simulink model "DrivetrainEv_3motor_VDBS"  (R2020a)
settings: configuration reference "Reference" (kept outside this file)
undefined symbols (not defined in the file): b, F0z, h, k, Ndiff_rear, VEH
libraries: vehdynlibsuspension x9, vehdynlibtire x8, autolibsharedcoupling x4, autolibcoupling x2, autolibutils x2, sharedtransform x2, autolibshareddiff x1, autolibshared x1, vehdynlibeom x1, vehdynlibtirecommon x1, vehdynlibsteering x1
(part 1 of 5)
settings Model: DataDictionary=System_Data_Dictionary.sldd  ModifiedByFormat=The MathWorks, Inc.  PauseTimes=10  OrderedModelArguments=off  Creator=The MathWorks, Inc.  LastModifiedBy=The MathWorks, Inc.
settings ConfigSetRef: SourceName=Reference

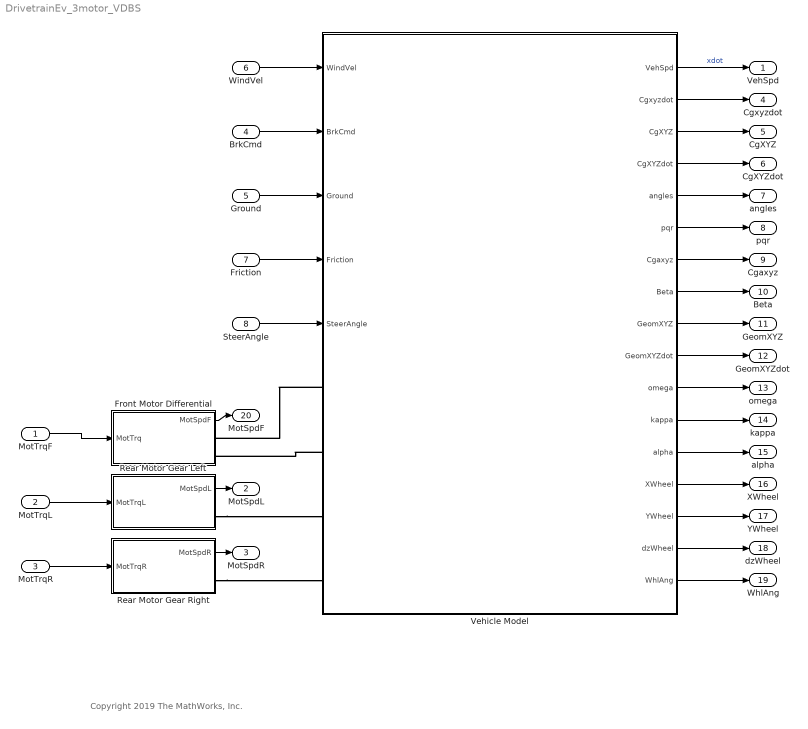
== system DrivetrainEv_3motor_VDBS ==
  note: Copyright 2019 The MathWorks, Inc.
  MotTrqF : Inport
  MotTrqL : Inport  Port=2
  MotTrqR : Inport  Port=3
  BrkCmd : Inport  Port=4
  Ground : Inport  Port=5
  WindVel : Inport  Port=6
  Friction : Inport  Port=7
  SteerAngle : Inport  Port=8
  Front Motor Differential : Subsystem  VariantControl=0
  Rear Motor Gear Left : Subsystem  VariantControl=0
  Rear Motor Gear Right : Subsystem  VariantControl=0
  Vehicle Model : Subsystem
  VehSpd : Outport  VectorParamsAs1DForOutWhenUnconnected=off
  MotSpdL : Outport  Port=2  VectorParamsAs1DForOutWhenUnconnected=off  BusOutputAsStruct=on
  MotSpdR : Outport  Port=3  VectorParamsAs1DForOutWhenUnconnected=off  BusOutputAsStruct=on
  Cgxyzdot : Outport  Port=4  VectorParamsAs1DForOutWhenUnconnected=off
  CgXYZ : Outport  Port=5  VectorParamsAs1DForOutWhenUnconnected=off
  CgXYZdot : Outport  Port=6  VectorParamsAs1DForOutWhenUnconnected=off
  angles : Outport  Port=7  VectorParamsAs1DForOutWhenUnconnected=off
  pqr : Outport  Port=8  VectorParamsAs1DForOutWhenUnconnected=off
  Cgaxyz : Outport  Port=9  VectorParamsAs1DForOutWhenUnconnected=off
  Beta : Outport  Port=10  VectorParamsAs1DForOutWhenUnconnected=off
  GeomXYZ : Outport  Port=11  VectorParamsAs1DForOutWhenUnconnected=off
  GeomXYZdot : Outport  Port=12  VectorParamsAs1DForOutWhenUnconnected=off
  omega : Outport  Port=13  PortDimensions=4  VectorParamsAs1DForOutWhenUnconnected=off
  kappa : Outport  Port=14  PortDimensions=4  VectorParamsAs1DForOutWhenUnconnected=off
  alpha : Outport  Port=15  PortDimensions=4  VectorParamsAs1DForOutWhenUnconnected=off
  XWheel : Outport  Port=16  VectorParamsAs1DForOutWhenUnconnected=off
  YWheel : Outport  Port=17  VectorParamsAs1DForOutWhenUnconnected=off
  dzWheel : Outport  Port=18  VectorParamsAs1DForOutWhenUnconnected=off
  WhlAng : Outport  Port=19  VectorParamsAs1DForOutWhenUnconnected=off
  MotSpdF : Outport  Port=20  VectorParamsAs1DForOutWhenUnconnected=off  BusOutputAsStruct=on
  wires:
  Rear Motor Gear Left/1(MotSpdL) -> MotSpdL/1
  Vehicle Model/12(kappa) -> kappa/1
  Vehicle Model/13(alpha) -> alpha/1
  Ground/1 -> Vehicle Model/3(Ground)
  Vehicle Model/14(XWheel) -> XWheel/1
  WindVel/1 -> Vehicle Model/1(WindVel)
  Vehicle Model/5(angles) -> angles/1
  Friction/1 -> Vehicle Model/4(Friction)
  SteerAngle/1 -> Vehicle Model/5(SteerAngle)
  Vehicle Model/8(Beta) -> Beta/1
  Vehicle Model/15(YWheel) -> YWheel/1
  Vehicle Model/17(WhlAng) -> WhlAng/1
  Vehicle Model/1(VehSpd) -> VehSpd/1  "xdot"
  Vehicle Model/10(GeomXYZdot) -> GeomXYZdot/1
  Vehicle Model/2(Cgxyzdot) -> Cgxyzdot/1
  Vehicle Model/4(CgXYZdot) -> CgXYZdot/1
  Vehicle Model/3(CgXYZ) -> CgXYZ/1
  Vehicle Model/7(Cgaxyz) -> Cgaxyz/1
  Vehicle Model/11(omega) -> omega/1
  Vehicle Model/9(GeomXYZ) -> GeomXYZ/1
  BrkCmd/1 -> Vehicle Model/2(BrkCmd)
  Vehicle Model/16(dzWheel) -> dzWheel/1
  Vehicle Model/6(pqr) -> pqr/1
  MotTrqL/1 -> Rear Motor Gear Left/1(MotTrqL)
  Rear Motor Gear Right/1(MotSpdR) -> MotSpdR/1
  MotTrqR/1 -> Rear Motor Gear Right/1(MotTrqR)
  Front Motor Differential/1(MotSpdF) -> MotSpdF/1
  MotTrqF/1 -> Front Motor Differential/1(MotTrq)
  connections:
  Vehicle Model/LConn1 -- Front Motor Differential/RConn1
  Vehicle Model/LConn2 -- Front Motor Differential/RConn2
  Rear Motor Gear Left/RConn1 -- Vehicle Model/LConn3
  Rear Motor Gear Right/RConn1 -- Vehicle Model/LConn4

== system DrivetrainEv_3motor_VDBS/Front Motor Differential ==
  MotTrq : Inport
  Axle Compliance : autolibsharedcoupling/Torsional Compliance  port_config=Two-way connection  extInfo=off  k=k  b=b  theta_o=theta_o  domega_o=domega_o  omega_c=omega_c  blkID=0  aMode=1
      settings: SourceProductName=Powertrain Blockset
  Axle Compliance1 : autolibsharedcoupling/Torsional Compliance  port_config=Two-way connection  extInfo=off  k=k  b=b  theta_o=theta_o  domega_o=domega_o  omega_c=omega_c  blkID=0  aMode=1
      settings: SourceProductName=Powertrain Blockset
  Open Differential : autolibshareddiff/Open Differential  DiffEffModelPopup=Constant  InterpMethod=Linear point-slope  extTamb=off  shaftSwitchMask=To the left of center-line  Ndiff=Ndiff_front  Jd=Jd  bd=bd  Jw1=Jw1  bw1=bw1  Jw2=Jw2  bw2=bw2  omegaw1o=omegaw1o  omegaw2o=omegaw2o  eta=1  eta_tbl=reshape([0.64 0.76 0.8 0.81 0.83 0.84 0.84 0.56 0.73 0.78 0.8 0.83 0.84 0.84 0.54 0.71 0.77 0.8 0.82 0.84 0.84 0.53 0.71 0.77 0.8 0.83 0.84 0.84 0.51 0.71 0.77 0.8 0.83 0.84 0.85 0.52 0.7 0.77 0.8 0.83 0.84 0.85 0.51 0.71 0.76 0.79 0.83 0.84 0.85 0.5 0.69 0.76 0.79 0.82 0.84 0.85 0.45 0.68 0.75 0.78 0.82 0.84 0.85 0.43 0.67 0.74 0.78 0.81 0.83 0.84 0.38 0.63 0.71 0.75 0.8 0.82 0.83 0.81 0.86 0.88 0.89 0.89 0.89 0.9 0.77 0.85 0.87 0.88 0.89 0.9 0.9 0.72 0.82 0.86 0.87 0.88 0.89 0.9 0.68 0.8 0.84 0.86 0.88 0.89 0.89 0.67 0.8 0.84 0.86 0.88 0.89 0.9 0.67 0.8 0.84 0.86 0.88 0.89 0.9 0.65 0.8 0.84 0.86 0.88 0.89 0.9 0.64 0.79 0.83 0.86 0.88 0.89 0.9 0.63 0.78 0.83 0.86 0.88 0.89 0.9 0.59 0.76 0.82 0.85 0.87 0.89 0.9 0.53 0.73 0.8 0.83 0.86 0.88 0.89], 7, 11, 2)  Trq_bpts=[25, 50, 75, 100, 150, 200, 250]  omega_bpts=[52.4 78.5 105 131 157 183 209 262 314 419 524]  Temp_bpts=[290 358]  Tamb=297.15  maxAbsSpd=5e3  aMode=1
      settings: SourceProductName=Powertrain Blockset
  Terminator6 : Terminator
  Two-Way Connection1 : TwoWayConnection
  Two-Way Connection3 : TwoWayConnection
  A1 : PMIOPort  Side=Right
  A2 : PMIOPort  Port=2  Side=Right
  MotSpdF : Outport  VectorParamsAs1DForOutWhenUnconnected=off
  wires:
  Open Differential/2 -> MotSpdF/1  "MotSpdF"
  Open Differential/4 -> Two-Way Connection3/1
  Open Differential/3 -> Two-Way Connection1/1
  Two-Way Connection1/1 -> Open Differential/2
  Open Differential/1 -> Terminator6/1  "Diff"
  Two-Way Connection3/1 -> Open Differential/3
  MotTrq/1 -> Open Differential/1
  connections:
  Axle Compliance/LConn1 -- Two-Way Connection1/RConn1
  Axle Compliance/RConn1 -- A1/RConn1
  Axle Compliance1/LConn1 -- Two-Way Connection3/RConn1
  A2/RConn1 -- Axle Compliance1/RConn1

== system DrivetrainEv_3motor_VDBS/Rear Motor Gear Left ==
  MotTrqL : Inport
  Axle Compliance : autolibsharedcoupling/Torsional Compliance  port_config=Two-way connection  extInfo=off  k=k  b=b  theta_o=theta_o  domega_o=domega_o  omega_c=omega_c  blkID=0  aMode=1
      settings: SourceProductName=Powertrain Blockset
  Gearbox : autolibcoupling/Gearbox  port_config=Simulink  input_config=Torque input - velocity output  DiffEffModelPopup=Constant  InterpMethod=Flat  dirSwitch=on  extTamb=off  N=Ndiff_rear  J1=J1  J2=J2  b1=b1_g  b2=b2_g  theta1_o=0  w1_o=w1_o  eta=1  eta_tbl=reshape([0.64 0.76 0.8 0.81 0.83 0.84 0.84 0.56 0.73 0.78 0.8 0.83 0.84 0.84 0.54 0.71 0.77 0.8 0.82 0.84 0.84 0.53 0.71 0.77 0.8 0.83 0.84 0.84 0.51 0.71 0.77 0.8 0.83 0.84 0.85 0.52 0.7 0.77 0.8 0.83 0.84 0.85 0.51 0.71 0.76 0.79 0.83 0.84 0.85 0.5 0.69 0.76 0.79 0.82 0.84 0.85 0.45 0.68 0.75 0.78 0.82 0.84 0.85 0.43 0.67 0.74 0.78 0.81 0.83 0.84 0.38 0.63 0.71 0.75 0.8 0.82 0.83 0.81 0.86 0.88 0.89 0.89 0.89 0.9 0.77 0.85 0.87 0.88 0.89 0.9 0.9 0.72 0.82 0.86 0.87 0.88 0.89 0.9 0.68 0.8 0.84 0.86 0.88 0.89 0.89 0.67 0.8 0.84 0.86 0.88 0.89 0.9 0.67 0.8 0.84 0.86 0.88 0.89 0.9 0.65 0.8 0.84 0.86 0.88 0.89 0.9 0.64 0.79 0.83 0.86 0.88 0.89 0.9 0.63 0.78 0.83 0.86 0.88 0.89 0.9 0.59 0.76 0.82 0.85 0.87 0.89 0.9 0.53 0.73 0.8 0.83 0.86 0.88 0.89], 7, 11, 2)  Trq_bpts=[25, 50, 75, 100, 150, 200, 250]  omega_bpts=[52.4 78.5 105 131 157 183 209 262 314 419 524]  Temp_bpts=[290 358]  Tamb=297.15  blkID=0
      settings: SourceProductBaseCode=PW
  Terminator6 : Terminator
  Two-Way Connection1 : TwoWayConnection
  AL : PMIOPort  Side=Right
  MotSpdL : Outport  VectorParamsAs1DForOutWhenUnconnected=off
  wires:
  Gearbox/2 -> MotSpdL/1
  MotTrqL/1 -> Gearbox/1
  Gearbox/3 -> Two-Way Connection1/1
  Two-Way Connection1/1 -> Gearbox/2
  Gearbox/1 -> Terminator6/1
  connections:
  Axle Compliance/LConn1 -- Two-Way Connection1/RConn1
  AL/RConn1 -- Axle Compliance/RConn1

== system DrivetrainEv_3motor_VDBS/Rear Motor Gear Right ==
  MotTrqR : Inport
  Axle Compliance : autolibsharedcoupling/Torsional Compliance  port_config=Two-way connection  extInfo=off  k=k  b=b  theta_o=theta_o  domega_o=domega_o  omega_c=omega_c  blkID=0  aMode=1
      settings: SourceProductName=Powertrain Blockset
  Gearbox : autolibcoupling/Gearbox  port_config=Simulink  input_config=Torque input - velocity output  DiffEffModelPopup=Constant  InterpMethod=Flat  dirSwitch=on  extTamb=off  N=Ndiff_rear  J1=J1  J2=J2  b1=b1_g  b2=b2_g  theta1_o=0  w1_o=w1_o  eta=1  eta_tbl=reshape([0.64 0.76 0.8 0.81 0.83 0.84 0.84 0.56 0.73 0.78 0.8 0.83 0.84 0.84 0.54 0.71 0.77 0.8 0.82 0.84 0.84 0.53 0.71 0.77 0.8 0.83 0.84 0.84 0.51 0.71 0.77 0.8 0.83 0.84 0.85 0.52 0.7 0.77 0.8 0.83 0.84 0.85 0.51 0.71 0.76 0.79 0.83 0.84 0.85 0.5 0.69 0.76 0.79 0.82 0.84 0.85 0.45 0.68 0.75 0.78 0.82 0.84 0.85 0.43 0.67 0.74 0.78 0.81 0.83 0.84 0.38 0.63 0.71 0.75 0.8 0.82 0.83 0.81 0.86 0.88 0.89 0.89 0.89 0.9 0.77 0.85 0.87 0.88 0.89 0.9 0.9 0.72 0.82 0.86 0.87 0.88 0.89 0.9 0.68 0.8 0.84 0.86 0.88 0.89 0.89 0.67 0.8 0.84 0.86 0.88 0.89 0.9 0.67 0.8 0.84 0.86 0.88 0.89 0.9 0.65 0.8 0.84 0.86 0.88 0.89 0.9 0.64 0.79 0.83 0.86 0.88 0.89 0.9 0.63 0.78 0.83 0.86 0.88 0.89 0.9 0.59 0.76 0.82 0.85 0.87 0.89 0.9 0.53 0.73 0.8 0.83 0.86 0.88 0.89], 7, 11, 2)  Trq_bpts=[25, 50, 75, 100, 150, 200, 250]  omega_bpts=[52.4 78.5 105 131 157 183 209 262 314 419 524]  Temp_bpts=[290 358]  Tamb=297.15  blkID=0
      settings: SourceProductBaseCode=PW
  Terminator6 : Terminator
  Two-Way Connection1 : TwoWayConnection
  AR : PMIOPort  Side=Right
  MotSpdR : Outport  VectorParamsAs1DForOutWhenUnconnected=off
  wires:
  Gearbox/1 -> Terminator6/1
  Two-Way Connection1/1 -> Gearbox/2
  Gearbox/3 -> Two-Way Connection1/1
  MotTrqR/1 -> Gearbox/1
  Gearbox/2 -> MotSpdR/1
  connections:
  AR/RConn1 -- Axle Compliance/RConn1
  Axle Compliance/LConn1 -- Two-Way Connection1/RConn1

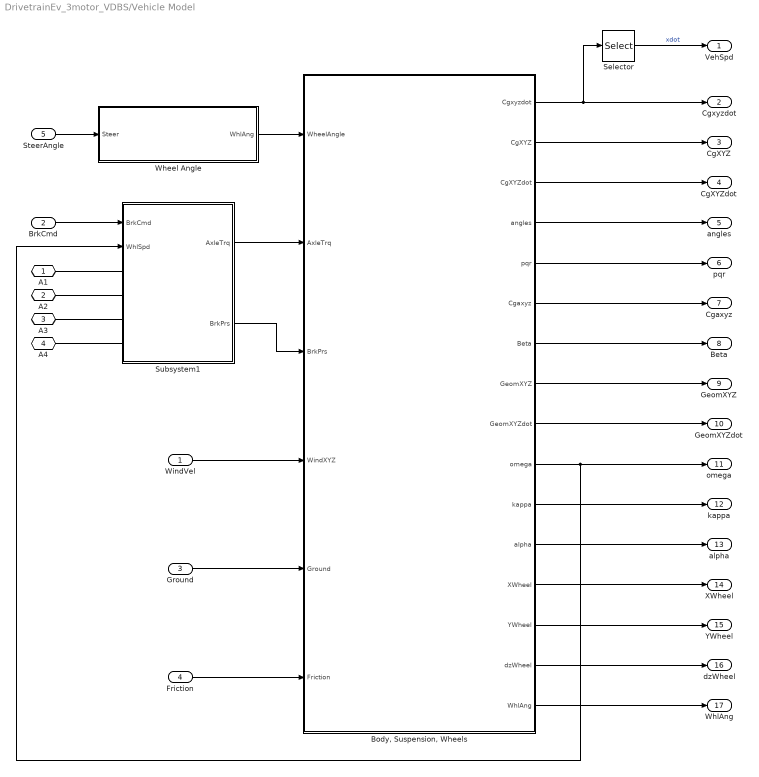
== system DrivetrainEv_3motor_VDBS/Vehicle Model ==
  WindVel : Inport
  BrkCmd : Inport  Port=2
  Ground : Inport  Port=3
  Friction : Inport  Port=4
  SteerAngle : Inport  Port=5
  "Body, Suspension, Wheels" : Subsystem  Variant=on  VariantControlMode=Label  LabelModeActiveChoice=1
  Selector : Selector  InputPortWidth=3  IndexOptions=Index vector (dialog)  Indices=1  OutputSizes=1
  Subsystem1 : Subsystem
  Wheel Angle : Subsystem
  A1 : PMIOPort  Side=Left
  A2 : PMIOPort  Port=2  Side=Left
  A3 : PMIOPort  Port=3  Side=Left
  A4 : PMIOPort  Port=4  Side=Left
  VehSpd : Outport  VectorParamsAs1DForOutWhenUnconnected=off
  Cgxyzdot : Outport  Port=2  VectorParamsAs1DForOutWhenUnconnected=off
  CgXYZ : Outport  Port=3  VectorParamsAs1DForOutWhenUnconnected=off
  CgXYZdot : Outport  Port=4  VectorParamsAs1DForOutWhenUnconnected=off
  angles : Outport  Port=5  VectorParamsAs1DForOutWhenUnconnected=off
  pqr : Outport  Port=6  VectorParamsAs1DForOutWhenUnconnected=off
  Cgaxyz : Outport  Port=7  VectorParamsAs1DForOutWhenUnconnected=off
  Beta : Outport  Port=8  VectorParamsAs1DForOutWhenUnconnected=off
  GeomXYZ : Outport  Port=9  VectorParamsAs1DForOutWhenUnconnected=off
  GeomXYZdot : Outport  Port=10  VectorParamsAs1DForOutWhenUnconnected=off
  omega : Outport  Port=11  PortDimensions=4  VectorParamsAs1DForOutWhenUnconnected=off
  kappa : Outport  Port=12  PortDimensions=4  VectorParamsAs1DForOutWhenUnconnected=off
  alpha : Outport  Port=13  PortDimensions=4  VectorParamsAs1DForOutWhenUnconnected=off
  XWheel : Outport  Port=14  VectorParamsAs1DForOutWhenUnconnected=off
  YWheel : Outport  Port=15  VectorParamsAs1DForOutWhenUnconnected=off
  dzWheel : Outport  Port=16  VectorParamsAs1DForOutWhenUnconnected=off
  WhlAng : Outport  Port=17  VectorParamsAs1DForOutWhenUnconnected=off
  wires:
  "Body, Suspension, Wheels"/10(omega) -> Subsystem1/2(WhlSpd), omega/1
  "Body, Suspension, Wheels"/8(GeomXYZ) -> GeomXYZ/1
  BrkCmd/1 -> Subsystem1/1(BrkCmd)
  "Body, Suspension, Wheels"/13(XWheel) -> XWheel/1
  "Body, Suspension, Wheels"/3(CgXYZdot) -> CgXYZdot/1
  "Body, Suspension, Wheels"/2(CgXYZ) -> CgXYZ/1
  "Body, Suspension, Wheels"/15(dzWheel) -> dzWheel/1
  "Body, Suspension, Wheels"/6(Cgaxyz) -> Cgaxyz/1
  "Body, Suspension, Wheels"/1(Cgxyzdot) -> Selector/1, Cgxyzdot/1
  "Body, Suspension, Wheels"/5(pqr) -> pqr/1
  "Body, Suspension, Wheels"/4(angles) -> angles/1
  "Body, Suspension, Wheels"/14(YWheel) -> YWheel/1
  "Body, Suspension, Wheels"/9(GeomXYZdot) -> GeomXYZdot/1
  "Body, Suspension, Wheels"/12(alpha) -> alpha/1
  "Body, Suspension, Wheels"/11(kappa) -> kappa/1
  "Body, Suspension, Wheels"/7(Beta) -> Beta/1
  "Body, Suspension, Wheels"/16(WhlAng) -> WhlAng/1
  Selector/1 -> VehSpd/1  "xdot"
  SteerAngle/1 -> Wheel Angle/1(Steer)
  WindVel/1 -> "Body, Suspension, Wheels"/4(WindXYZ)
  Wheel Angle/1(WhlAng) -> "Body, Suspension, Wheels"/1(WheelAngle)
  Ground/1 -> "Body, Suspension, Wheels"/5(Ground)
  Friction/1 -> "Body, Suspension, Wheels"/6(Friction)
  Subsystem1/2(BrkPrs) -> "Body, Suspension, Wheels"/3(BrkPrs)
  Subsystem1/1(AxleTrq) -> "Body, Suspension, Wheels"/2(AxleTrq)
  connections:
  Subsystem1/LConn1 -- A1/RConn1
  A2/RConn1 -- Subsystem1/LConn2
  A3/RConn1 -- Subsystem1/LConn3
  A4/RConn1 -- Subsystem1/LConn4

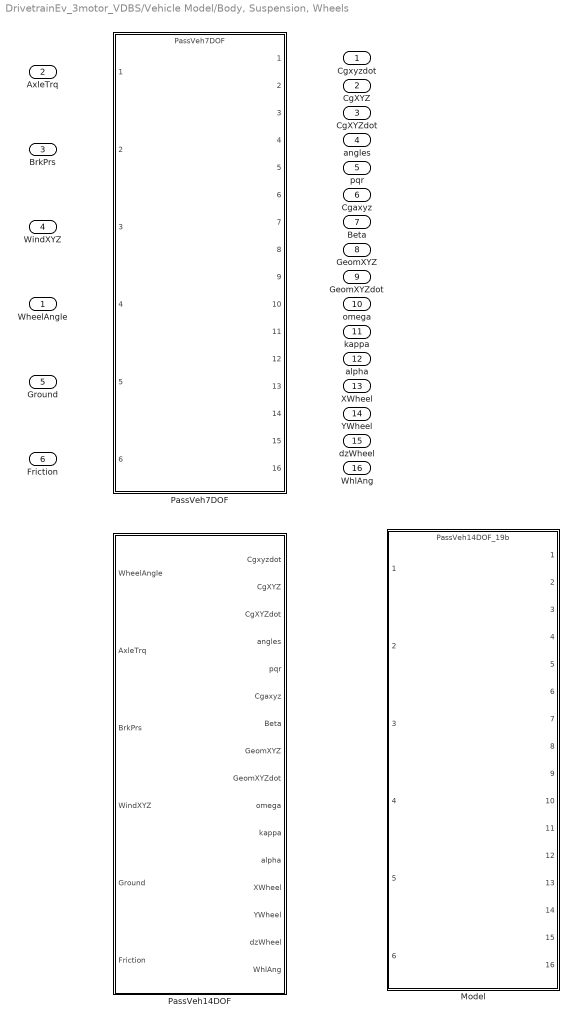
== system DrivetrainEv_3motor_VDBS/Vehicle Model/Body, Suspension, Wheels ==
  WheelAngle : Inport
  AxleTrq : Inport  Port=2
  BrkPrs : Inport  Port=3
  WindXYZ : Inport  Port=4
  Ground : Inport  Port=5
  Friction : Inport  Port=6
  Model : ModelReference  ModelNameDialog=PassVeh14DOF_19b.slx  SimulationMode=Normal  VariantControl=Choice  ModelReferenceVersion=1.318
  PassVeh14DOF : Subsystem  VariantControl=1
  PassVeh7DOF : ModelReference  DisableCoverage=on  ModelNameDialog=PassVeh7DOF  VariantControl=0  ModelReferenceVersion=1.140
  Cgxyzdot : Outport  VectorParamsAs1DForOutWhenUnconnected=off
  CgXYZ : Outport  Port=2  VectorParamsAs1DForOutWhenUnconnected=off
  CgXYZdot : Outport  Port=3  VectorParamsAs1DForOutWhenUnconnected=off
  angles : Outport  Port=4  VectorParamsAs1DForOutWhenUnconnected=off
  pqr : Outport  Port=5  VectorParamsAs1DForOutWhenUnconnected=off
  Cgaxyz : Outport  Port=6  VectorParamsAs1DForOutWhenUnconnected=off
  Beta : Outport  Port=7  VectorParamsAs1DForOutWhenUnconnected=off
  GeomXYZ : Outport  Port=8  VectorParamsAs1DForOutWhenUnconnected=off
  GeomXYZdot : Outport  Port=9  VectorParamsAs1DForOutWhenUnconnected=off
  omega : Outport  Port=10  PortDimensions=4  VectorParamsAs1DForOutWhenUnconnected=off
  kappa : Outport  Port=11  PortDimensions=4  VectorParamsAs1DForOutWhenUnconnected=off
  alpha : Outport  Port=12  PortDimensions=4  VectorParamsAs1DForOutWhenUnconnected=off
  XWheel : Outport  Port=13  VectorParamsAs1DForOutWhenUnconnected=off
  YWheel : Outport  Port=14  VectorParamsAs1DForOutWhenUnconnected=off
  dzWheel : Outport  Port=15  VectorParamsAs1DForOutWhenUnconnected=off
  WhlAng : Outport  Port=16  VectorParamsAs1DForOutWhenUnconnected=off

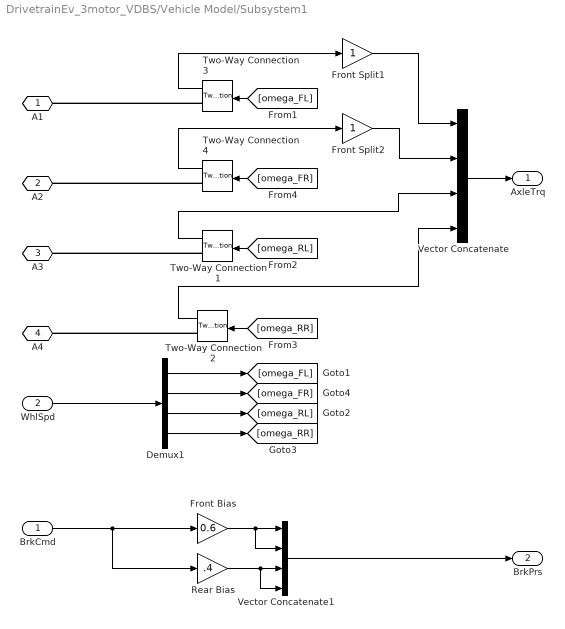
== system DrivetrainEv_3motor_VDBS/Vehicle Model/Subsystem1 ==
  BrkCmd : Inport
  WhlSpd : Inport  Port=2
  Demux1 : Demux
  Front Bias : Gain  Gain=0.6
  Front Split1 : Gain
  Front Split2 : Gain
  Rear Bias : Gain  Gain=.4
  Two-Way Connection{1..4} (4 alike) : TwoWayConnection
  Vector Concatenate : Concatenate  NumInputs=4
  Vector Concatenate1 : Concatenate  NumInputs=4
  A1 : PMIOPort  Side=Left
  A2 : PMIOPort  Port=2  Side=Left
  A3 : PMIOPort  Port=3  Side=Left
  A4 : PMIOPort  Port=4  Side=Left
  AxleTrq : Outport  VectorParamsAs1DForOutWhenUnconnected=off
  BrkPrs : Outport  Port=2  VectorParamsAs1DForOutWhenUnconnected=off
  wires:
  [omega_FL] -> Two-Way Connection3/1
  Vector Concatenate/1 -> AxleTrq/1
  WhlSpd/1 -> Demux1/1
  Demux1/1 -> [omega_FL]
  Demux1/3 -> [omega_RL]
  Demux1/4 -> [omega_RR]
  Two-Way Connection3/1 -> Front Split1/1
  [omega_FR] -> Two-Way Connection4/1
  Demux1/2 -> [omega_FR]
  Two-Way Connection4/1 -> Front Split2/1
  Front Split1/1 -> Vector Concatenate/1
  Front Split2/1 -> Vector Concatenate/2
  Vector Concatenate1/1 -> BrkPrs/1
  BrkCmd/1 -> Front Bias/1, Rear Bias/1
  Front Bias/1 -> Vector Concatenate1/2, Vector Concatenate1/1
  Rear Bias/1 -> Vector Concatenate1/4, Vector Concatenate1/3
  [omega_RL] -> Two-Way Connection1/1
  [omega_RR] -> Two-Way Connection2/1
  Two-Way Connection1/1 -> Vector Concatenate/3
  Two-Way Connection2/1 -> Vector Concatenate/4
  connections:
  Two-Way Connection3/RConn1 -- A1/RConn1
  Two-Way Connection4/RConn1 -- A2/RConn1
  Two-Way Connection2/RConn1 -- A4/RConn1
  Two-Way Connection1/RConn1 -- A3/RConn1

== system DrivetrainEv_3motor_VDBS/Vehicle Model/Wheel Angle ==
  Steer : Inport
  Ground3 : Ground
  Kinematic Steering : vehdynlibsteering/Kinematic Steering  StrgType=Ackerman  StrgRatioType=Constant  Loc=Front  NrmlFctr=1  TrckWdth=1.922  WhlBase=(1.515+1.504)  Db=0  StrgRng=3*pi  StrgAngBpts="[-6.2832   -5.0265   -3.7699   -2.5133   -1.2566         0    1.2566    2.5133    3.7699    5.0265    6.2832]"  StrgRatioTbl=|  StrgRatio=18  StrgArmLngth=0.1  RckCsLngth=0.5  TieRodLngth=0.248128028933392  D=0.2  PnnRadius=0.0057  PnnRadiusTbl="[0.0055    0.0055    0.0056    0.0057    0.0057    0.0057    0.0057    0.0057    0.0056    0.0055    0.0055]"  RodLngth=0.1  ParaArmLngth=0.9  aMode=2
      | [13.5000   13.3750   13.2500   13.1250   13.0000   13.0000   13.0000   13.1250   13.2500   13.3750   13.5000
      | ]
  Terminator : Terminator
  Vector Concatenate : Concatenate
  Vector Concatenate1 : Concatenate
  Vector Concatenate2 : Concatenate
  WhlAng : Outport  Unit=rad  VectorParamsAs1DForOutWhenUnconnected=off
  wires:
  Kinematic Steering/3 -> Vector Concatenate/2
  Ground3/1 -> Vector Concatenate2/2, Vector Concatenate2/1
  Vector Concatenate1/1 -> WhlAng/1
  Vector Concatenate/1 -> Vector Concatenate1/1  "FrontWheelAngles"
  Kinematic Steering/1 -> Terminator/1
  Kinematic Steering/2 -> Vector Concatenate/1
  Vector Concatenate2/1 -> Vector Concatenate1/2  "RearWheelAngles"
  Steer/1 -> Kinematic Steering/1

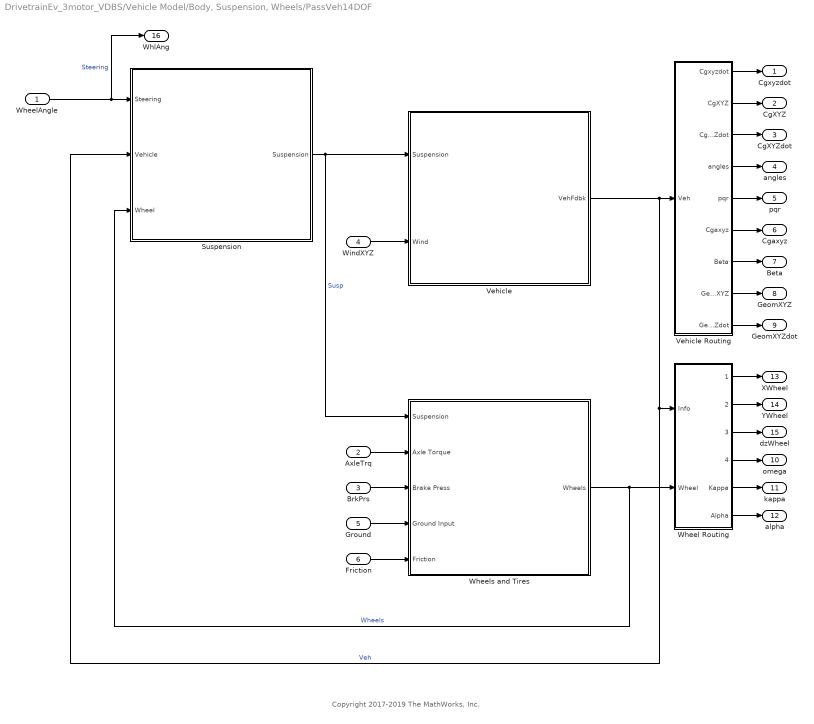
== system DrivetrainEv_3motor_VDBS/Vehicle Model/Body, Suspension, Wheels/PassVeh14DOF ==
  note: Copyright 2017-2019 The MathWorks, Inc.
  WheelAngle : Inport  Unit=rad
  AxleTrq : Inport  Port=2  Unit=N*m
  BrkPrs : Inport  Port=3
  WindXYZ : Inport  Port=4  Unit=m/s  PortDimensions=3
  Ground : Inport  Port=5  Unit=m
  Friction : Inport  Port=6  Unit=1
  Suspension : Subsystem  Variant=on  VariantControlMode=Label  LabelModeActiveChoice=2
      mask Display:
      | switch str2num(get_param(gcb,'ActiveVariant'))
      |     case 1
      |         image('suspdw.png');
      |     case 2
      |         image([imread('suspindmap.png');imread('suspsamap.png')]);
      |     case 3
      |          image([imread('suspmacp.png');imread('suspsacoil.png')]);
      |     case 4
      |          image('suspmacp.png');
      |     case 5
      |          image('suspindmap.png');
      | end
  Vehicle : Subsystem
      mask Display: image('6dofcar.png');
  Vehicle Routing : Subsystem
  Wheel Routing : Subsystem
  Wheels and Tires : Subsystem
      mask Display: image('wheel3dof.png')
  Cgxyzdot : Outport  VectorParamsAs1DForOutWhenUnconnected=off
  CgXYZ : Outport  Port=2  VectorParamsAs1DForOutWhenUnconnected=off
  CgXYZdot : Outport  Port=3  VectorParamsAs1DForOutWhenUnconnected=off
  angles : Outport  Port=4  VectorParamsAs1DForOutWhenUnconnected=off
  pqr : Outport  Port=5  VectorParamsAs1DForOutWhenUnconnected=off
  Cgaxyz : Outport  Port=6  VectorParamsAs1DForOutWhenUnconnected=off
  Beta : Outport  Port=7  VectorParamsAs1DForOutWhenUnconnected=off
  GeomXYZ : Outport  Port=8  VectorParamsAs1DForOutWhenUnconnected=off
  GeomXYZdot : Outport  Port=9  VectorParamsAs1DForOutWhenUnconnected=off
  omega : Outport  Port=10  PortDimensions=4  VectorParamsAs1DForOutWhenUnconnected=off
  kappa : Outport  Port=11  PortDimensions=4  VectorParamsAs1DForOutWhenUnconnected=off
  alpha : Outport  Port=12  PortDimensions=4  VectorParamsAs1DForOutWhenUnconnected=off
  XWheel : Outport  Port=13  VectorParamsAs1DForOutWhenUnconnected=off
  YWheel : Outport  Port=14  VectorParamsAs1DForOutWhenUnconnected=off
  dzWheel : Outport  Port=15  PortDimensions=4  VectorParamsAs1DForOutWhenUnconnected=off
  WhlAng : Outport  Port=16  VectorParamsAs1DForOutWhenUnconnected=off
  wires:
  Wheel Routing/3(ZWheel) -> dzWheel/1
  Wheel Routing/4(Omega) -> omega/1
  Vehicle Routing/5(pqr) -> pqr/1
  Wheel Routing/5(Kappa) -> kappa/1
  Vehicle Routing/4(angles) -> angles/1
  Vehicle Routing/3(CgXYZdot) -> CgXYZdot/1
  WheelAngle/1 -> WhlAng/1, Suspension/1(Steering)  "Steering"
  Vehicle Routing/1(Cgxyzdot) -> Cgxyzdot/1
  Vehicle Routing/9(GeomXYZdot) -> GeomXYZdot/1
  Ground/1 -> Wheels and Tires/4(Ground Input)
  Wheel Routing/1(XWheel) -> XWheel/1
  Wheel Routing/2(YWheel) -> YWheel/1
  AxleTrq/1 -> Wheels and Tires/2(Axle Torque)
  Vehicle Routing/8(GeomXYZ) -> GeomXYZ/1
  Vehicle Routing/7(Beta) -> Beta/1
  Wheels and Tires/1(Wheels) -> Suspension/3(Wheel), Wheel Routing/2(Wheel)  "Wheels"
  Vehicle Routing/6(Cgaxyz) -> Cgaxyz/1
  Wheel Routing/6(Alpha) -> alpha/1
  Vehicle Routing/2(CgXYZ) -> CgXYZ/1
  BrkPrs/1 -> Wheels and Tires/3(Brake Press)
  WindXYZ/1 -> Vehicle/2(Wind)
  Vehicle/1(VehFdbk) -> Suspension/2(Vehicle), Wheel Routing/1(Info), Vehicle Routing/1(Veh)  "Veh"
  Friction/1 -> Wheels and Tires/5(Friction)
  Suspension/1(Suspension) -> Wheels and Tires/1(Suspension), Vehicle/1(Suspension)  "Susp"

== system DrivetrainEv_3motor_VDBS/Vehicle Model/Body, Suspension, Wheels/PassVeh14DOF/Suspension ==
  Steering : Inport
  Vehicle : Inport  Port=2
  Wheel : Inport  Port=3
  Double Wishbone Suspension : Subsystem  VariantControl=1
      mask Display: image('suspdw.png');
  Independent Mapped Front Suspension Mapped Solid Axle Rear Suspension : Subsystem  VariantControl=2
      mask Display: image([imread('suspindmap.png');imread('suspsamap.png')]);
  MacPherson Front Suspension Mapped Independent Rear Suspension : Subsystem  VariantControl=6
      mask Display: image([imread('suspmacp.png');imread('suspsacoil.png')]);
  MacPherson Front Suspension Solid Axle Rear Suspension : Subsystem  VariantControl=3
      mask Display: image([imread('suspmacp.png');imread('suspsacoil.png')]);
  MacPherson Suspension : Subsystem  VariantControl=4
      mask Display: image('suspmacp.png');
  Mapped Suspension : Subsystem  VariantControl=5
      mask Display: image('suspindmap.png');
  Suspension : Outport  VectorParamsAs1DForOutWhenUnconnected=off

== system DrivetrainEv_3motor_VDBS/Vehicle Model/Body, Suspension, Wheels/PassVeh14DOF/Vehicle ==
  Suspension : Inport
  Wind : Inport  Port=2
  Variant Subsystem : Subsystem  Variant=on  VariantControlMode=Label  LabelModeActiveChoice=1
  VehFdbk : Outport  VectorParamsAs1DForOutWhenUnconnected=off
  wires:
  Variant Subsystem/1(VehFdbk) -> VehFdbk/1  "VehFdbk"
  Wind/1 -> Variant Subsystem/2(Wind)
  Suspension/1 -> Variant Subsystem/1(Suspension)

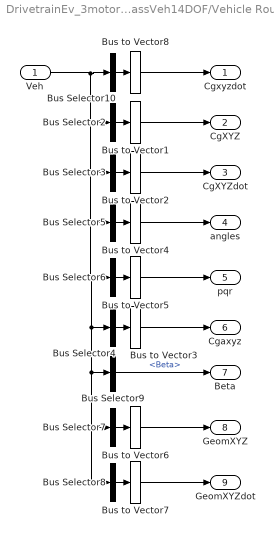
== system DrivetrainEv_3motor_VDBS/Vehicle Model/Body, Suspension, Wheels/PassVeh14DOF/Vehicle Routing ==
  Veh : Inport
  Bus Selector10 : BusSelector  OutputSignals=BdyFrm.Cg.Vel.xdot,BdyFrm.Cg.Vel.ydot,BdyFrm.Cg.Vel.zdot  OutputAsBus=on
  Bus Selector2 : BusSelector  OutputSignals=InertFrm.Cg.Disp.X,InertFrm.Cg.Disp.Y,InertFrm.Cg.Disp.Z  OutputAsBus=on
  Bus Selector3 : BusSelector  OutputSignals=InertFrm.Cg.Vel.Xdot,InertFrm.Cg.Vel.Ydot,InertFrm.Cg.Vel.Zdot  OutputAsBus=on
  Bus Selector4 : BusSelector  OutputSignals=BdyFrm.Cg.Acc.ax,BdyFrm.Cg.Acc.ay,BdyFrm.Cg.Acc.az  OutputAsBus=on
  Bus Selector5 : BusSelector  OutputSignals=InertFrm.Cg.Ang.phi,InertFrm.Cg.Ang.theta,InertFrm.Cg.Ang.psi  OutputAsBus=on
  Bus Selector6 : BusSelector  OutputSignals=BdyFrm.Cg.AngVel.p,BdyFrm.Cg.AngVel.q,BdyFrm.Cg.AngVel.r  OutputAsBus=on
  Bus Selector7 : BusSelector  OutputSignals=InertFrm.Geom.Disp.X,InertFrm.Geom.Disp.Y,InertFrm.Geom.Disp.Z  OutputAsBus=on
  Bus Selector8 : BusSelector  OutputSignals=InertFrm.Geom.Vel.Xdot,InertFrm.Geom.Vel.Ydot,InertFrm.Geom.Vel.Zdot  OutputAsBus=on
  Bus Selector9 : BusSelector  OutputSignals=BdyFrm.Geom.Ang.Beta
  Bus to Vector{1..8} (8 alike) : BusToVector
  Cgxyzdot : Outport  VectorParamsAs1DForOutWhenUnconnected=off
  CgXYZ : Outport  Port=2  VectorParamsAs1DForOutWhenUnconnected=off
  CgXYZdot : Outport  Port=3  VectorParamsAs1DForOutWhenUnconnected=off
  angles : Outport  Port=4  VectorParamsAs1DForOutWhenUnconnected=off
  pqr : Outport  Port=5  VectorParamsAs1DForOutWhenUnconnected=off
  Cgaxyz : Outport  Port=6  VectorParamsAs1DForOutWhenUnconnected=off
  Beta : Outport  Port=7  VectorParamsAs1DForOutWhenUnconnected=off
  GeomXYZ : Outport  Port=8  VectorParamsAs1DForOutWhenUnconnected=off
  GeomXYZdot : Outport  Port=9  VectorParamsAs1DForOutWhenUnconnected=off
  wires:
  Bus Selector3/1 -> Bus to Vector2/1
  Bus to Vector1/1 -> CgXYZ/1
  Bus to Vector5/1 -> pqr/1
  Bus Selector5/1 -> Bus to Vector4/1
  Bus Selector6/1 -> Bus to Vector5/1
  Bus to Vector4/1 -> angles/1
  Bus to Vector8/1 -> Cgxyzdot/1
  Bus Selector2/1 -> Bus to Vector1/1
  Bus Selector8/1 -> Bus to Vector7/1
  Bus to Vector6/1 -> GeomXYZ/1
  Bus Selector9/1 -> Beta/1  "<Beta>"
  Bus Selector4/1 -> Bus to Vector3/1
  Bus Selector10/1 -> Bus to Vector8/1
  Bus to Vector7/1 -> GeomXYZdot/1
  Bus to Vector3/1 -> Cgaxyz/1
  Bus Selector7/1 -> Bus to Vector6/1
  Bus to Vector2/1 -> CgXYZdot/1
  Veh/1 -> Bus Selector8/1, Bus Selector7/1, Bus Selector9/1, Bus Selector4/1, Bus Selector6/1, Bus Selector5/1, Bus Selector3/1, Bus Selector2/1, Bus Selector10/1

== system DrivetrainEv_3motor_VDBS/Vehicle Model/Body, Suspension, Wheels/PassVeh14DOF/Wheel Routing ==
  Info : Inport
  Wheel : Inport  Port=2
  Bus Selector : BusSelector  OutputSignals=InertFrm.FrntAxl.Lft.Disp.Y,InertFrm.FrntAxl.Rght.Disp.Y,InertFrm.RearAxl.Lft.Disp.Y,InertFrm.RearAxl.Rght.Disp.Y
  Bus Selector1 : BusSelector  OutputSignals=InertFrm.FrntAxl.Lft.Disp.X,InertFrm.FrntAxl.Rght.Disp.X,InertFrm.RearAxl.Lft.Disp.X,InertFrm.RearAxl.Rght.Disp.X
  Bus Selector2 : BusSelector  OutputSignals=TireFrame.z,TireFrame.Omega,TireFrame.Kappa,TireFrame.Alpha
  Bus Selector3 : BusSelector  OutputSignals=InertFrm.FrntAxl.Lft.Disp.Z,InertFrm.FrntAxl.Rght.Disp.Z,InertFrm.RearAxl.Lft.Disp.Z,InertFrm.RearAxl.Rght.Disp.Z
  Bus Selector4 : BusSelector  OutputSignals=BdyFrm.FrntAxl.Lft.Disp.z,BdyFrm.FrntAxl.Rght.Disp.z,BdyFrm.RearAxl.Lft.Disp.z,BdyFrm.RearAxl.Rght.Disp.z
  Subtract : Sum  Inputs=-+-
  Vector Concatenate{1..4} (4 alike) : Concatenate  NumInputs=4
  XWheel : Outport  Unit=m  VectorParamsAs1DForOutWhenUnconnected=off
  YWheel : Outport  Port=2  Unit=m  VectorParamsAs1DForOutWhenUnconnected=off
  ZWheel : Outport  Port=3  PortDimensions=4  VectorParamsAs1DForOutWhenUnconnected=off
  Omega : Outport  Port=4  PortDimensions=4  VectorParamsAs1DForOutWhenUnconnected=off
  Kappa : Outport  Port=5  PortDimensions=4  VectorParamsAs1DForOutWhenUnconnected=off
  Alpha : Outport  Port=6  PortDimensions=4  VectorParamsAs1DForOutWhenUnconnected=off
  wires:
  Bus Selector1/4 -> Vector Concatenate2/4  "<X>"
  Bus Selector/1 -> Vector Concatenate1/1  "<Y>"
  Bus Selector1/3 -> Vector Concatenate2/3  "<X>"
  Bus Selector/4 -> Vector Concatenate1/4  "<Y>"
  Bus Selector1/2 -> Vector Concatenate2/2  "<X>"
  Bus Selector/3 -> Vector Concatenate1/3  "<Y>"
  Bus Selector/2 -> Vector Concatenate1/2  "<Y>"
  Vector Concatenate1/1 -> YWheel/1
  Bus Selector1/1 -> Vector Concatenate2/1  "<X>"
  Vector Concatenate2/1 -> XWheel/1
  Bus Selector2/1 -> Subtract/3  "<z>"
  Bus Selector2/2 -> Omega/1  "<Omega>"
  Bus Selector2/3 -> Kappa/1  "<Kappa>"
  Bus Selector2/4 -> Alpha/1  "<Alpha>"
  Wheel/1 -> Bus Selector2/1
  Subtract/1 -> ZWheel/1
  Info/1 -> Bus Selector1/1, Bus Selector4/1, Bus Selector3/1, Bus Selector/1
  Bus Selector3/2 -> Vector Concatenate3/2  "<Z>"
  Bus Selector3/3 -> Vector Concatenate3/3  "<Z>"
  Bus Selector3/4 -> Vector Concatenate3/4  "<Z>"
  Bus Selector3/1 -> Vector Concatenate3/1  "<Z>"
  Vector Concatenate3/1 -> Subtract/2
  Vector Concatenate4/1 -> Subtract/1
  Bus Selector4/1 -> Vector Concatenate4/1  "<z>"
  Bus Selector4/4 -> Vector Concatenate4/4  "<z>"
  Bus Selector4/3 -> Vector Concatenate4/3  "<z>"
  Bus Selector4/2 -> Vector Concatenate4/2  "<z>"

== system DrivetrainEv_3motor_VDBS/Vehicle Model/Body, Suspension, Wheels/PassVeh14DOF/Wheels and Tires ==
  Suspension : Inport
  Axle Torque : Inport  Port=2
  Brake Press : Inport  Port=3  Unit=Pa
  Ground Input : Inport  Port=4
  Friction : Inport  Port=5  PortDimensions=4
  Bus Selector1 : BusSelector  OutputSignals=Whl.Ang,Whl.F,Whl.AngVel,Whl.xdot,Whl.ydot
  Constant3 : Constant  Value=zeros(4,1)
  Cont LPF : autolibutils/Cont LPF  wc=100*2*pi  aMode=2
      settings: SourceProductBaseCode=PW
  Cont LPF1 : autolibutils/Cont LPF  wc=100*2*pi  aMode=2
      settings: SourceProductBaseCode=PW
  Manual Switch6 : ManualSwitch
  Matrix Concatenate : Concatenate  NumInputs=3  Mode=Multidimensional array
  Reshape1 : Reshape
  Reshape2 : Reshape
  Saturation : Saturate  UpperLimit=inf  LowerLimit=-10*9.81*2000  ZeroCross=off
  Selector : Selector  NumberOfDimensions=2  InputPortWidth=3  IndexOptions=Index vector (dialog),Select all  Indices=[3],1  OutputSizes=1,1
  Selector1 : Selector  NumberOfDimensions=2  InputPortWidth=1  IndexOptions=Index vector (dialog),Select all  Indices=[3],1  OutputSizes=1,1
  Selector2 : Selector  NumberOfDimensions=2  InputPortWidth=3  IndexOptions=Index vector (dialog),Select all  Indices=3,1  OutputSizes=1,1
  Selector3 : Selector  NumberOfDimensions=2  InputPortWidth=3  IndexOptions=Index vector (dialog),Select all  Indices=1,1  OutputSizes=1,1
  Terminator{,1,3..5} (5 alike) : Terminator
  VDBS : Subsystem  VariantControl=0
  Wheels : Outport  VectorParamsAs1DForOutWhenUnconnected=off
  wires:
  VDBS/1(WhlAng) -> Wheels/1  "Wheels"
  Bus Selector1/2 -> Selector/1  "<F>"
  VDBS/2(FrntAxlF) -> Terminator/1
  VDBS/3(RearAxlF) -> Terminator1/1
  VDBS/4(Omega) -> Terminator3/1
  VDBS/5(Mz) -> Terminator4/1
  Selector1/1 -> Reshape1/1
  Matrix Concatenate/1 -> VDBS/7(VehVel)
  Axle Torque/1 -> VDBS/3(AxleTrq)
  Selector2/1 -> VDBS/1(WheelAng)  "Wheel Angles"
  Constant3/1 -> Manual Switch6/1
  Manual Switch6/1 -> VDBS/2(CamberAng)  "Camber Angles"
  Selector/1 -> Reshape2/1
  Saturation/1 -> VDBS/5(Fz)
  Ground Input/1 -> VDBS/8(Ground Level)
  VDBS/7(SuspWhlVz) -> Matrix Concatenate/3  "zdot"
  Bus Selector1/1 -> Cont LPF1/1  "<Ang>"
  Selector3/1 -> Manual Switch6/2  "Camber Angles"
  Suspension/1 -> Bus Selector1/1
  Bus Selector1/4 -> Matrix Concatenate/1  "<xdot>"
  Bus Selector1/5 -> Matrix Concatenate/2  "<ydot>"
  VDBS/6(SuspWhlPz) -> Terminator5/1  "z"
  Reshape2/1 -> Cont LPF/1
  Bus Selector1/3 -> Selector1/1  "<AngVel>"
  Reshape1/1 -> VDBS/6(r)
  Brake Press/1 -> VDBS/4(BrkPrs)
  Friction/1 -> VDBS/9(Friction)
  Cont LPF/1 -> Saturation/1
  Cont LPF1/1 -> Selector3/1, Selector2/1

== system DrivetrainEv_3motor_VDBS/Vehicle Model/Body, Suspension, Wheels/PassVeh14DOF/Suspension/Double Wishbone Suspension ==
  Wheel : Inport
  Steering : Inport  Port=2
  Vehicle : Inport  Port=3
  Bus Creator1 : BusCreator  Inputs=5
  Bus Creator2 : BusCreator  Inputs=2
  Bus Creator3 : BusCreator  Inputs=2
  Bus Creator4 : BusCreator  Inputs=6
  Bus Selector : BusSelector  OutputSignals=z,Re,zdot,Fx,Fy,M
  Bus Selector1 : BusSelector  OutputSignals=P,V
  Independent Suspension – Double Wishbone : vehdynlibsuspension/Independent Suspension - Double Wishbone  ActiveDampEn=off  NumAxl=2  NumTracksByAxl=[2 2]  StrgEnByAxl=[1 0]  AntiSwayEnByAxl=[1 0]  TrackNumVec="[1  2  1  2]"  AxleNumVec="[1  1  2  2]"  SuspTypesByAxle="[1  1]"  SuspImage=suspdw.png  IdealSuspEn=on  IdealSuspAxles="[1  2]"  Kz=Kz  F0z=F0z  Cz=Cz  Hmax=Hmax  f_act_susp_cz=[10000 10000;10000 10000]  f_act_susp_duty_bpt=[0 1]  f_act_susp_zdot_bpt=[-1 1]  Toe=0.  RollStrgSlp=0.  ToeStrgSlp=0.  Caster=0.  CasterHslp=0.  CasterStrgSlp=0.  Camber=0.  CamberHslp=0.  CamberStrgSlp=0.  StrgHgtSlp=0.1432  MappedSuspEn=off  MappedSuspAxles="[1  2]"  f_susp_axl_bp=[1 2]  f_susp_dz_bp=[-0.15 -0.14 -0.13 -0.12 -0.11 -0.10 -0.09 -0.08 -0.07 -0.06 -0.05 -0.04 -0.03 -0.02 -0.01 0.00 0.01 0.02 0.03 0.04 0.05 0.06 0.07 0.08 0.09 0.10 0.11 0.12 0.13 0.14 0.15]  f_susp_dzdot_bp=[-0.15 -0.14 -0.13 -0.12 -0.11 -0.10 -0.09 -0.08 -0.07 -0.06 -0.05 -0.04 -0.03 -0.02 -0.01 0.00 0.01 0.02 0.03 0.04 0.05 0.06 0.07 0.08 0.09 0.10 0.11 0.12 0.13 0.14 0.15]  f_susp_fmz=zeros(31,31,61,2,4)  f_susp_geom=zeros(31,61,2,3)  f_susp_strgdelta_bp=[-30,-29,-28,-27,-26,-25,-24,-23,-22,-21,-20,-19,-18,-17,-16,-15,-14,-13,-12,-11,-10,-9,-8,-7,-6,-5,-4,-3,-2,-1,0,1,2,3,4,5,6,7,8,9,10,11,12,13,14,15,16,17,18,19,20,21,22,23,24,25,26,27,28,29,30]  AntiSwayR=0.2  AntiSwayNtrlAng=0.5236  AntiSwayTrsK=8e2
      settings: SourceProductBaseCode=VE
  Selector1 : Selector  NumberOfDimensions=2  IndexOptions=Index vector (dialog),Select all  Indices=1,1  OutputSizes=1,1
  Selector2 : Selector  NumberOfDimensions=2  IndexOptions=Index vector (dialog),Select all  Indices=2,1  OutputSizes=1,1
  Steer Rate Adapter : Subsystem
  Steering Adapter : Subsystem
  Terminator : Terminator
  Vehicle Adapter : Subsystem
  Wheel  Adapter : Subsystem
  Suspension : Outport  VectorParamsAs1DForOutWhenUnconnected=off
  wires:
  Bus Creator3/1 -> Suspension/1
  Steering Adapter/1(StrgAng) -> Independent Suspension – Double Wishbone/9
  Independent Suspension – Double Wishbone/1 -> Terminator/1  "Susp"
  Wheel  Adapter/6(Re) -> Bus Creator4/6
  Bus Selector1/1 -> Independent Suspension – Double Wishbone/7  "<P>"
  Wheel  Adapter/2(WhlFy) -> Bus Creator4/2  "Fy"
  Wheel/1 -> Wheel  Adapter/1(Wheels)
  Steer Rate Adapter/1(AngVel) -> Bus Creator1/5  "AngVel"
  Bus Creator4/1 -> Bus Selector/1
  Bus Creator2/1 -> Bus Creator3/1  "Veh"
  Independent Suspension – Double Wishbone/5 -> Selector2/1, Selector1/1  "V"
  Selector2/1 -> Bus Creator1/3  "ydot"
  Bus Selector1/2 -> Independent Suspension – Double Wishbone/8  "<V>"
  Independent Suspension – Double Wishbone/2 -> Bus Creator2/1  "F"
  Bus Selector/2 -> Independent Suspension – Double Wishbone/2  "<Re>"
  Wheel  Adapter/5(M) -> Bus Creator4/5  "M"
  Bus Selector/4 -> Independent Suspension – Double Wishbone/4  "<Fx>"
  Independent Suspension – Double Wishbone/4 -> Bus Creator1/1  "F"
  Steering/1 -> Steering Adapter/1(Steer)
  Selector1/1 -> Bus Creator1/2  "xdot"
  Independent Suspension – Double Wishbone/3 -> Bus Creator2/2  "M"
  Vehicle Adapter/1(VehSusp) -> Bus Selector1/1
  Wheel  Adapter/4(zdot) -> Bus Creator4/4
  Vehicle/1 -> Steer Rate Adapter/1(Veh), Vehicle Adapter/1(Veh)
  Bus Selector/6 -> Independent Suspension – Double Wishbone/6  "<M>"
  Bus Selector/5 -> Independent Suspension – Double Wishbone/5  "<Fy>"
  Bus Selector/1 -> Independent Suspension – Double Wishbone/1  "<z>"
  Wheel  Adapter/3(z) -> Bus Creator4/3
  Independent Suspension – Double Wishbone/6 -> Bus Creator1/4  "Ang"
  Bus Creator1/1 -> Bus Creator3/2  "Whl"
  Wheel  Adapter/1(WhlFx) -> Bus Creator4/1  "Fx"
  Bus Selector/3 -> Independent Suspension – Double Wishbone/3  "<zdot>"

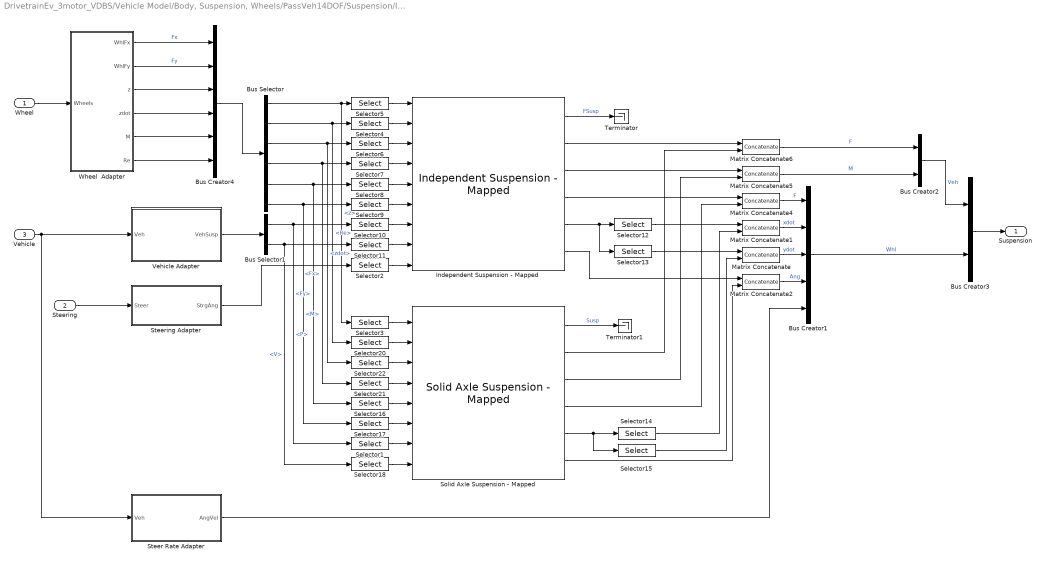
== system DrivetrainEv_3motor_VDBS/Vehicle Model/Body, Suspension, Wheels/PassVeh14DOF/Suspension/Independent Mapped Front Suspension Mapped Solid Axle Rear Suspension ==
  Wheel : Inport
  Steering : Inport  Port=2
  Vehicle : Inport  Port=3
  Bus Creator1 : BusCreator  Inputs=5
  Bus Creator2 : BusCreator  Inputs=2
  Bus Creator3 : BusCreator  Inputs=2
  Bus Creator4 : BusCreator  Inputs=6
  Bus Selector : BusSelector  OutputSignals=z,Re,zdot,Fx,Fy,M
  Bus Selector1 : BusSelector  OutputSignals=P,V
  Independent Suspension - Mapped : vehdynlibsuspension/Independent Suspension - Mapped  NumAxl=1  NumTracksByAxl=2  StrgEnByAxl=1  AntiSwayEnByAxl=1  TrackNumVec="[1  2]"  AxleNumVec="[1  1]"  SuspTypesByAxle=[2]  SuspImage=suspindmap.png  IdealSuspEn=off  IdealSuspAxles="[1  2]"  Kz=64370  F0z=9810  Cz=10000  Hmax=0.5  Toe=2  RollStrgSlp=-13  ToeStrgSlp=0.01  Caster=4  CasterHslp=-13  CasterStrgSlp=0.01  Camber=4  CamberHslp=-13  CamberStrgSlp=0.01  StrgHgtSlp=0.0025  MappedSuspEn=on  MappedSuspAxles=[1]  f_susp_axl_bp=[1 2]  f_susp_dz_bp=f_susp_dz_bp  f_susp_dzdot_bp=f_susp_dzdot_bp  f_susp_fmz=f_susp_fmz  f_susp_geom=f_susp_geom  f_susp_strgdelta_bp=f_susp_strgdelta_bp  NDFLookupOutType=1:4  NDGLookupOutType=1:3  AntiSwayR=0.2  AntiSwayNtrlAng=0.5236  AntiSwayTrsK=8e2
      link override For each track and axle combination calculate suspension forces and moments/Suspension/Suspension Angle Calculations: OverrideUsingVariant=MappedSteeringEnabled
      link override For each track and axle combination calculate suspension forces and moments/Suspension/Z axis suspension characteristic: OverrideUsingVariant=MappedSuspension
      settings: SourceProductBaseCode=VE
  Matrix Concatenate{,1..2,4..6} (6 alike) : Concatenate  Mode=Multidimensional array  ConcatenateDimension=2
  Selector1 : Selector  NumberOfDimensions=2  IndexOptions=Select all,Index vector (dialog)  Indices=[1 2],[3 4]  OutputSizes=1,1
  Selector10 : Selector  NumberOfDimensions=2  IndexOptions=Select all,Index vector (dialog)  Indices=[1 2],[1 2]  OutputSizes=1,1
  Selector11 : Selector  NumberOfDimensions=2  IndexOptions=Select all,Index vector (dialog)  Indices=[1 2],[1 2]  OutputSizes=1,1
  Selector12 : Selector  NumberOfDimensions=2  InputPortWidth=3  IndexOptions=Index vector (dialog),Select all  Indices=1,1  OutputSizes=1,1
  Selector13 : Selector  NumberOfDimensions=2  InputPortWidth=3  IndexOptions=Index vector (dialog),Select all  Indices=2,1  OutputSizes=1,1
  Selector14 : Selector  NumberOfDimensions=2  InputPortWidth=3  IndexOptions=Index vector (dialog),Select all  Indices=1,1  OutputSizes=1,1
  Selector15 : Selector  NumberOfDimensions=2  InputPortWidth=3  IndexOptions=Index vector (dialog),Select all  Indices=2,1  OutputSizes=1,1
  Selector{3,16,20..22} (5 alike) : Selector  IndexOptions=Index vector (dialog)  Indices=[3 4]  OutputSizes=1
  Selector17 : Selector  NumberOfDimensions=2  IndexOptions=Select all,Index vector (dialog)  Indices=[1 2],[3 4]  OutputSizes=1,1
  Selector18 : Selector  NumberOfDimensions=2  IndexOptions=Select all,Index vector (dialog)  Indices=[1 2],[3 4]  OutputSizes=1,1
  Selector{2,4..8} (6 alike) : Selector  IndexOptions=Index vector (dialog)  Indices=[1 2]  OutputSizes=1
  Selector9 : Selector  NumberOfDimensions=2  IndexOptions=Select all,Index vector (dialog)  Indices=[1 2],[1 2]  OutputSizes=1,1
  Solid Axle Suspension - Mapped : vehdynlibsuspension/Solid Axle Suspension - Mapped  NumAxl=1  NumTracksByAxl=2  StrgEnByAxl=0  TrackNumVec="[1  2]"  AxleNumVec="[1  1]"  SuspTypesByAxle=[2]  SuspImage=suspsamap.png  AxlIxx=AxlIxx  AxlM=AxlM  TrackCoords=[0 0;VEH.TrackWidth*[-1 1]/2;0 0]  SuspCoords=[0 0;VEH.TrackWidth*[-1 1]/2;0 0]  KzWhlAxl=KzWhlAxl  F0zWhlAxl=F0zWhlAxl  CzWhlAxl=CzWhlAxl  IdealSuspEn=off  IdealSuspAxles="[1  2]"  Kz=64370  F0z=9810  Cz=10000  Hmax=0.5  Toe=2  RollStrgSlp=-13  ToeStrgSlp=0.01  Caster=4  CasterHslp=-13  CasterStrgSlp=0.01  Camber=4  CamberHslp=-13  CamberStrgSlp=0.01  StrgHgtSlp=0.0025  MappedSuspEn=on  MappedSuspAxles=[1]  f_susp_axl_bp=[1 2]  f_susp_dz_bp=f_susp_dz_bp  f_susp_dzdot_bp=f_susp_dzdot_bp  f_susp_fmz=f_susp_fmz  f_susp_geom=f_susp_geom  f_susp_strgdelta_bp=f_susp_strgdelta_bp  NDFLookupOutType=1:4  NDGLookupOutType=1:3
      link override For each track and axle combination calculate suspension forces and moments/Suspension/Suspension Angle Calculations: OverrideUsingVariant=MappedSteeringEnabled
      link override For each track and axle combination calculate suspension forces and moments/Suspension/Z axis suspension characteristic: OverrideUsingVariant=MappedSuspension
      settings: SourceProductBaseCode=VE
  Steer Rate Adapter : Subsystem
  Steering Adapter : Subsystem
  Terminator : Terminator
  Terminator1 : Terminator
  Vehicle Adapter : Subsystem
  Wheel  Adapter : Subsystem
  Suspension : Outport  VectorParamsAs1DForOutWhenUnconnected=off
  wires:
  Solid Axle Suspension - Mapped/5 -> Selector15/1, Selector14/1
  Selector22/1 -> Solid Axle Suspension - Mapped/3
  Bus Selector/3 -> Selector22/1, Selector6/1  "<zdot>"
  Solid Axle Suspension - Mapped/4 -> Matrix Concatenate4/2
  Solid Axle Suspension - Mapped/1 -> Terminator1/1  "Susp"
  Selector12/1 -> Matrix Concatenate1/1
  Selector7/1 -> Independent Suspension - Mapped/4
  Selector18/1 -> Solid Axle Suspension - Mapped/8
  Selector13/1 -> Matrix Concatenate/1
  Selector14/1 -> Matrix Concatenate1/2
  Selector21/1 -> Solid Axle Suspension - Mapped/4
  Vehicle/1 -> Steer Rate Adapter/1(Veh), Vehicle Adapter/1(Veh)
  Wheel  Adapter/4(zdot) -> Bus Creator4/4
  Solid Axle Suspension - Mapped/3 -> Matrix Concatenate5/2
  Selector1/1 -> Solid Axle Suspension - Mapped/7
  Matrix Concatenate4/1 -> Bus Creator1/1  "F"
  Selector16/1 -> Solid Axle Suspension - Mapped/5
  Matrix Concatenate5/1 -> Bus Creator2/2  "M"
  Independent Suspension - Mapped/4 -> Matrix Concatenate4/1
  Selector4/1 -> Independent Suspension - Mapped/2
  Selector10/1 -> Independent Suspension - Mapped/7
  Selector9/1 -> Independent Suspension - Mapped/6
  Wheel  Adapter/3(z) -> Bus Creator4/3
  Solid Axle Suspension - Mapped/2 -> Matrix Concatenate6/2
  Wheel/1 -> Wheel  Adapter/1(Wheels)
  Selector5/1 -> Independent Suspension - Mapped/1
  Independent Suspension - Mapped/3 -> Matrix Concatenate5/1
  Selector8/1 -> Independent Suspension - Mapped/5
  Independent Suspension - Mapped/2 -> Matrix Concatenate6/1
  Independent Suspension - Mapped/6 -> Matrix Concatenate2/1
  Selector20/1 -> Solid Axle Suspension - Mapped/2
  Independent Suspension - Mapped/1 -> Terminator/1  "FSusp"
  Bus Creator2/1 -> Bus Creator3/1  "Veh"
  Bus Selector/4 -> Selector7/1, Selector21/1  "<Fx>"
  Independent Suspension - Mapped/5 -> Selector12/1, Selector13/1
  Matrix Concatenate2/1 -> Bus Creator1/4  "Ang"
  Wheel  Adapter/2(WhlFy) -> Bus Creator4/2  "Fy"
  Bus Creator4/1 -> Bus Selector/1
  Selector17/1 -> Solid Axle Suspension - Mapped/6
  Selector2/1 -> Independent Suspension - Mapped/9
  Wheel  Adapter/5(M) -> Bus Creator4/5
  Matrix Concatenate/1 -> Bus Creator1/3  "ydot"
  Steering/1 -> Steering Adapter/1(Steer)
  Matrix Concatenate1/1 -> Bus Creator1/2  "xdot"
  Selector15/1 -> Matrix Concatenate/2
  Selector3/1 -> Solid Axle Suspension - Mapped/1
  Bus Selector1/2 -> Selector11/1, Selector18/1  "<V>"
  Vehicle Adapter/1(VehSusp) -> Bus Selector1/1
  Steering Adapter/1(StrgAng) -> Selector2/1
  Selector6/1 -> Independent Suspension - Mapped/3
  Bus Selector/6 -> Selector9/1, Selector17/1  "<M>"
  Wheel  Adapter/1(WhlFx) -> Bus Creator4/1  "Fx"
  Selector11/1 -> Independent Suspension - Mapped/8
  Wheel  Adapter/6(Re) -> Bus Creator4/6
  Matrix Concatenate6/1 -> Bus Creator2/1  "F"
  Bus Selector1/1 -> Selector10/1, Selector1/1  "<P>"
  Solid Axle Suspension - Mapped/6 -> Matrix Concatenate2/2
  Bus Selector/1 -> Selector3/1, Selector5/1  "<z>"
  Bus Selector/5 -> Selector8/1, Selector16/1  "<Fy>"
  Bus Creator1/1 -> Bus Creator3/2  "Whl"
  Bus Creator3/1 -> Suspension/1
  Bus Selector/2 -> Selector20/1, Selector4/1  "<Re>"
  Steer Rate Adapter/1(AngVel) -> Bus Creator1/5
